simulink model "Tp3"  (R2017b)
settings: Solver=ode23s  StartTime=0.0  StopTime=10.0  RelTol=1e-3
InitFcn:
  | Tp3_data
values from neighbouring files (symbols this model uses):
  Cr = 0    [MCC_constants.m]    (also in Td2.m; Tp3_data.m)
  J = 3.2284E-6    (= 3.2284e-06)    [MCC_constants.m]    (also in ProjetGiesData.m = 0.5; Td2.m = 0.28; Tp3_data.m = 0.2)
  L = 2.75E-6    (= 2.75e-06)    [MCC_constants.m]    (also in Td2.m = 0.0016; Tp3_data.m = 0.012161)
  p = 3    [Tp3_data.m]
  Phif = K/p    (= 0.3)    [Tp3_data.m]
  PI = 3.1415    [ProjetGiesData.m]    (also in Tp3_data.m)
  psi = PI/4    (= 0.785375)    [Tp3_data.m]
  R = 4    [MCC_constants.m]    (also in Td2.m = 0.13; Tp3_data.m = 0.895)
  U0 = 220    [Tp3_data.m]
settings Model: Creator=Table2  LastModifiedBy=Table2

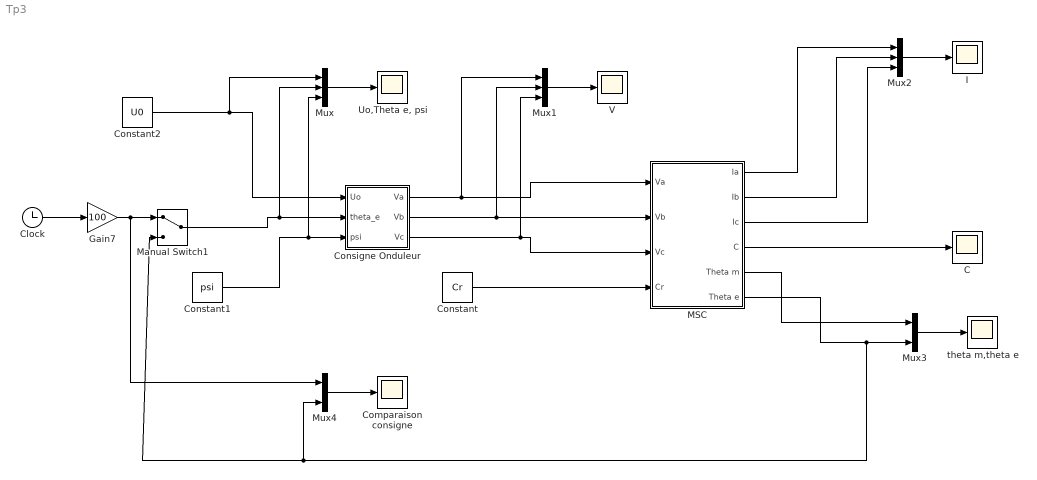
== system Tp3 ==
  C : Scope
  Clock : Clock
  Comparaison consigne : Scope
  "Consigne Onduleur " : Subsystem
  Constant : Constant  Value=Cr
  Constant1 : Constant  Value=psi
  Constant2 : Constant  Value=U0
  Gain7 : Gain  Gain=100
  I : Scope
  "MSC " : Subsystem
  Manual Switch1 : ManualSwitch
  Mux : Mux  Inputs=3
  Mux1 : Mux  Inputs=3
  Mux2 : Mux  Inputs=3
  Mux3 : Mux  Inputs=2
  Mux4 : Mux  Inputs=2
  "Uo,Theta e, psi" : Scope
  V : Scope
  theta m,theta e : Scope
  wires:
  Constant/1 -> "MSC "/4(Cr)
  Constant1/1 -> Mux/3, "Consigne Onduleur "/3("psi ")
  Constant2/1 -> Mux/1, "Consigne Onduleur "/1("Uo ")
  Clock/1 -> Gain7/1
  Gain7/1 -> Mux4/1, Manual Switch1/1
  Manual Switch1/1 -> Mux/2, "Consigne Onduleur "/2("theta_e ")
  Mux/1 -> "Uo,Theta e, psi"/1
  "Consigne Onduleur "/2(Vb) -> Mux1/2, "MSC "/2(Vb)
  "Consigne Onduleur "/3(Vc) -> Mux1/3, "MSC "/3(Vc)
  "Consigne Onduleur "/1(Va) -> Mux1/1, "MSC "/1(Va)
  Mux1/1 -> V/1
  "MSC "/3(Ic) -> Mux2/3
  "MSC "/2(Ib) -> Mux2/2
  "MSC "/1(Ia) -> Mux2/1
  Mux2/1 -> I/1
  "MSC "/4(C) -> C/1
  Mux3/1 -> theta m,theta e/1
  "MSC "/5("Theta m ") -> Mux3/1
  "MSC "/6("Theta e ") -> Mux4/2, Manual Switch1/2, Mux3/2
  Mux4/1 -> Comparaison consigne/1

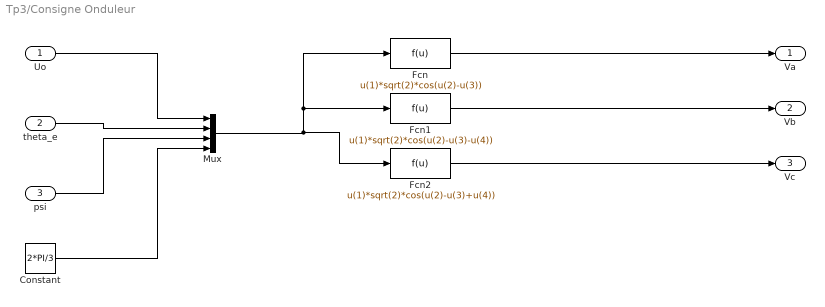
== system Tp3/Consigne Onduleur  ==
  "Uo " : Inport
  "theta_e " : Inport  Port=2
  "psi " : Inport  Port=3
  Constant : Constant  Value=2*PI/3
  Fcn : Fcn  Expr=u(1)*sqrt(2)*cos(u(2)-u(3))
  Fcn1 : Fcn  Expr=u(1)*sqrt(2)*cos(u(2)-u(3)-u(4))
  Fcn2 : Fcn  Expr=u(1)*sqrt(2)*cos(u(2)-u(3)+u(4))
  Mux : Mux
  Va : Outport
  Vb : Outport  Port=2
  Vc : Outport  Port=3
  wires:
  Fcn/1 -> Va/1
  "theta_e "/1 -> Mux/2
  "psi "/1 -> Mux/3
  "Uo "/1 -> Mux/1
  Mux/1 -> Fcn2/1, Fcn1/1, Fcn/1
  Constant/1 -> Mux/4
  Fcn1/1 -> Vb/1
  Fcn2/1 -> Vc/1

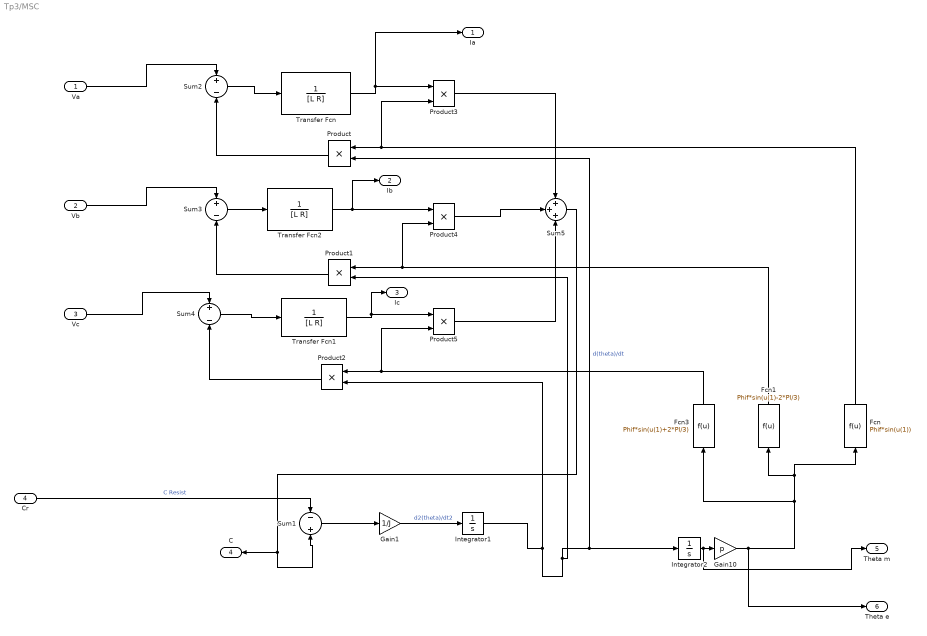
== system Tp3/MSC  ==
  Va : Inport
  Vb : Inport  Port=2
  Vc : Inport  Port=3
  Cr : Inport  Port=4
  Fcn : Fcn  Expr=Phif*sin(u(1))
  Fcn1 : Fcn  Expr=Phif*sin(u(1)-2*PI/3)
  Fcn3 : Fcn  Expr=Phif*sin(u(1)+2*PI/3)
  Gain1 : Gain  Gain=1/J
  Gain10 : Gain  Gain=p
  Integrator1 : Integrator
  Integrator2 : Integrator
  Product{,1..5} (6 alike) : Product
  Sum1 : Sum  Inputs=-|+
  Sum2 : Sum  Inputs=+-
  Sum3 : Sum  Inputs=+|-
  Sum4 : Sum  Inputs=+|-
  Sum5 : Sum  Inputs=+++
  Transfer Fcn : TransferFcn  Denominator=[L R]
  Transfer Fcn1 : TransferFcn  Denominator=[L R]
  Transfer Fcn2 : TransferFcn  Denominator=[L R]
  Ia : Outport
  Ib : Outport  Port=2
  Ic : Outport  Port=3
  C : Outport  Port=4
  "Theta m " : Outport  Port=5
  "Theta e " : Outport  Port=6
  wires:
  Cr/1 -> Sum1/1  "C Resist"
  Sum1/1 -> Gain1/1
  Gain1/1 -> Integrator1/1  "d2(theta)/dt2"
  Integrator2/1 -> "Theta m "/1, Gain10/1
  Va/1 -> Sum2/1
  Vb/1 -> Sum3/1
  Vc/1 -> Sum4/1
  Sum4/1 -> Transfer Fcn1/1
  Sum3/1 -> Transfer Fcn2/1
  Sum2/1 -> Transfer Fcn/1
  Gain10/1 -> Fcn3/1, Fcn1/1, Fcn/1, "Theta e "/1
  Fcn/1 -> Product3/2, Product/1
  Product/1 -> Sum2/2
  Fcn1/1 -> Product4/2, Product1/1
  Product1/1 -> Sum3/2
  Fcn3/1 -> Product5/2, Product2/1
  Product2/1 -> Sum4/2
  Integrator1/1 -> Product2/2, Product1/2, Product/2, Integrator2/1  "d(theta)/dt"
  Sum5/1 -> C/1, Sum1/2
  Transfer Fcn1/1 -> Ic/1, Product5/1
  Transfer Fcn2/1 -> Ib/1, Product4/1
  Transfer Fcn/1 -> Ia/1, Product3/1
  Product3/1 -> Sum5/1
  Product4/1 -> Sum5/2
  Product5/1 -> Sum5/3
